simulink model "ROPOD_Control_SIM"  (R2017b)
settings: Solver=VariableStepAuto  StartTime=0.0  StopTime=inf  RelTol=1e-3
values from neighbouring files (symbols this model uses):
  AgentNumber = 1    [init_model.m]
  FFtheta_intia = 0    [init_model.m]
  FFxy_mass = 0*80    (= 0)    [init_model.m]
  flock_FFtheta_friction = 50    [init_model.m]
  flock_FFxy_friction = 100    [init_model.m]
  I_fhz_ddelta_cntr = 0    [init_model.m]
  I_fhz_dtheta_cntr = 0.3    [init_model.m]
  I_fhz_dtheta_flock_cntr = 0.1    [init_model.m]
  I_fhz_dvarphi_cntr = 0    [init_model.m]
  I_fhz_dxdy_cntr = 0.25    [init_model.m]
  I_fhz_dxdy_flock_cntr = 0.1    [init_model.m]
  K_gain_ddelta_cntr = 0.1    [init_model.m]
  K_gain_dtheta_cntr = 150    [init_model.m]
  K_gain_dtheta_flock_cntr = 100    [init_model.m]
  K_gain_dvarphi_cntr = 0.05    [init_model.m]
  K_gain_dxdy_cntr = 200    [init_model.m]
  K_gain_dxdy_flock_cntr = 200    [init_model.m]
  LL_wp_fhz_ddelta_cntr = 2    [init_model.m]
  LL_wp_fhz_dtheta_cntr = 20    [init_model.m]
  LL_wp_fhz_dtheta_flock_cntr = 20    [init_model.m]
  LL_wp_fhz_dvarphi_cntr = 10    [init_model.m]
  LL_wp_fhz_dxdy_cntr = 20    [init_model.m]
  LL_wp_fhz_dxdy_flock_cntr = 20    [init_model.m]
  LL_wz_fhz_ddelta_cntr = 2    [init_model.m]
  LL_wz_fhz_dtheta_cntr = 20    [init_model.m]
  LL_wz_fhz_dtheta_flock_cntr = 20    [init_model.m]
  LL_wz_fhz_dvarphi_cntr = 2    [init_model.m]
  LL_wz_fhz_dxdy_cntr = 20    [init_model.m]
  LL_wz_fhz_dxdy_flock_cntr = 20    [init_model.m]
  LPF_fhz_ddelta_cntr = 50    [init_model.m]
  LPF_fhz_ddelta_meas = 50    [init_model.m]
  LPF_fhz_dtheta_cntr = 100    [init_model.m]
  LPF_fhz_dtheta_flock_cntr = 40    [init_model.m]
  LPF_fhz_dvarphi_cntr = 50    [init_model.m]
  LPF_fhz_dvarphi_meas = 50    [init_model.m]
  LPF_fhz_dxdy_cntr = 100    [init_model.m]
  LPF_fhz_dxdy_flock_cntr = 40    [init_model.m]
  max_flock_acc_theta = 0.5    [init_model.m]
  max_flock_acc_xy = 0.5    [init_model.m]
  max_flock_vel_theta = 1.0    (= 1)    [init_model.m]
  max_flock_vel_xy = 1.0    (= 1)    [init_model.m]
  max_hw_tau = 7.0    (= 7)    [init_model.m]
  max_ropod_acc_theta = 1.6    [init_model.m]
  max_ropod_acc_xy = 2.0    (= 2)    [init_model.m]
  max_ropod_sw_force = 500    [init_model.m]
  max_ropod_sw_tau = 250    [init_model.m]
  max_ropod_vel_theta = 1.6    [init_model.m]
  max_ropod_vel_xy = 2.0    (= 2)    [init_model.m]
  max_sw_current = 10    [init_model.m]
  Nagents = 2    [init_model.m]
  Nwheels = 4    [Jqwl_numeric_function.m]    (also in S_matrix.m; extract_kinmodel_parameters.m; init_model.m; tau_optimal_dist_vec_fun.m)
  pivot_offs_sws = [0.0243    0.4689    0.3384    5.9050]    [init_model.m]
  ropod_kinmodel_pv = struct2array(ropod_kinmodel_param)    [set_ropod_KinModparams.m]
  ropod_position_inflock = [-1 0 3.1416]    [init_model.m]
  SW_COM1_ENABLE1 = hex2dec('0001')    [init_model.m]
  SW_COM1_ENABLE2 = hex2dec('0002')    [init_model.m]
  SW_COM1_MODE_TORQUE = bitshift(hex2dec('0000'),2)    [init_model.m]
  SW_COM1_MODE_VELOCITY = bitshift(hex2dec('0002'),2)    [init_model.m]
  SW_COM1_USE_TS = hex2dec('8000')    [init_model.m]
  sw_tau_2_current = 1/motor_physical_parameters.torqueconstant.value    [init_model.m]
  Tinit = 2    [init_model.m]
  Ts = 0.001    [init_model.m]
  Ts_MPC = 0.01    [init_model.m]
  Tsflck = 0.01    [init_model.m]
undefined symbols (not defined in the file or in its folder): acc_limit, accmax, b_cx, b_cy, b_rx, bus_size, comp_enable, Desired, DiscIntNeverNeededParam, Fcgain, gdis, k_cx, k_cy, live_tuning, m_robot, Nominal, Nominal_x, Nominal_y, offsets, portwidth, sizes, types, vel_limit, vmax1, vmax2
libraries: simulink x90, cstblocks x66, dspsigops x12, dspnetwork x4
(part 4 of 8)

== system ROPOD_Control_SIM/RopodTorqueDistribution/wheel vel cntr/Wheels Velocity controller ==
  dvarphi_error : Inport
  ena_w : Inport  Port=2
  platform_dvarphi_cntr_param : Inport  Port=3
  reset_int : Inport  Port=4
  Demux : Demux  Outputs=8
  Demux1 : Demux
  G_I_LL_LPF Controller1 : Subsystem
  G_I_LL_LPF Controller2 : Subsystem
  G_I_LL_LPF Controller3 : Subsystem
  G_I_LL_LPF Controller4 : Subsystem
  G_I_LL_LPF Controller5 : Subsystem
  G_I_LL_LPF Controller6 : Subsystem
  G_I_LL_LPF Controller7 : Subsystem
  G_I_LL_LPF Controller8 : Subsystem
  Mux : Mux  Inputs=8
  Mux1 : Mux  Inputs=8
  Product9 : Product
  varphi_tau_setp : Outport
  wires:
  Product9/1 -> Demux/1
  dvarphi_error/1 -> Product9/1
  [reset_int_cntr] -> G_I_LL_LPF Controller1/3(reset_integrator)
  Demux/1 -> G_I_LL_LPF Controller1/2(In)
  [param_dvarphi_cntr] -> G_I_LL_LPF Controller1/1(param)
  platform_dvarphi_cntr_param/1 -> [param_dvarphi_cntr]
  reset_int/1 -> [reset_int_cntr]
  [param_dvarphi_cntr] -> G_I_LL_LPF Controller2/1(param)
  [reset_int_cntr] -> G_I_LL_LPF Controller2/3(reset_integrator)
  Demux/2 -> G_I_LL_LPF Controller2/2(In)
  [reset_int_cntr] -> G_I_LL_LPF Controller4/3(reset_integrator)
  Demux/3 -> G_I_LL_LPF Controller3/2(In)
  Demux/4 -> G_I_LL_LPF Controller4/2(In)
  [param_dvarphi_cntr] -> G_I_LL_LPF Controller4/1(param)
  [param_dvarphi_cntr] -> G_I_LL_LPF Controller3/1(param)
  [reset_int_cntr] -> G_I_LL_LPF Controller3/3(reset_integrator)
  [param_dvarphi_cntr] -> G_I_LL_LPF Controller5/1(param)
  Demux/8 -> G_I_LL_LPF Controller8/2(In)
  [param_dvarphi_cntr] -> G_I_LL_LPF Controller7/1(param)
  [param_dvarphi_cntr] -> G_I_LL_LPF Controller8/1(param)
  [reset_int_cntr] -> G_I_LL_LPF Controller8/3(reset_integrator)
  [param_dvarphi_cntr] -> G_I_LL_LPF Controller6/1(param)
  [reset_int_cntr] -> G_I_LL_LPF Controller7/3(reset_integrator)
  Demux/6 -> G_I_LL_LPF Controller6/2(In)
  Demux/7 -> G_I_LL_LPF Controller7/2(In)
  [reset_int_cntr] -> G_I_LL_LPF Controller6/3(reset_integrator)
  [reset_int_cntr] -> G_I_LL_LPF Controller5/3(reset_integrator)
  Demux/5 -> G_I_LL_LPF Controller5/2(In)
  G_I_LL_LPF Controller1/1(Out) -> Mux/1
  G_I_LL_LPF Controller2/1(Out) -> Mux/2
  G_I_LL_LPF Controller4/1(Out) -> Mux/4
  G_I_LL_LPF Controller3/1(Out) -> Mux/3
  G_I_LL_LPF Controller5/1(Out) -> Mux/5
  G_I_LL_LPF Controller6/1(Out) -> Mux/6
  G_I_LL_LPF Controller7/1(Out) -> Mux/7
  G_I_LL_LPF Controller8/1(Out) -> Mux/8
  Mux/1 -> varphi_tau_setp/1
  ena_w/1 -> Demux1/1
  Demux1/1 -> Mux1/2, Mux1/1
  Demux1/2 -> Mux1/4, Mux1/3
  Demux1/3 -> Mux1/6, Mux1/5
  Demux1/4 -> Mux1/8, Mux1/7
  Mux1/1 -> Product9/2

== system ROPOD_Control_SIM/RopodVelocityController/Platorm Velocity controller/G_I_LL_LPF Controller_X ==
  param : Inport
  In : Inport  Port=2
  reset_integrator : Inport  Port=3
  Bus Selector : BusSelector  OutputSignals=P_gain,I_freq_hz,LL_zero_fhz,LL_pole_fhz,LPF_fhz
  Discrete Varying Lowpass3 : cstblocks/Linear Parameter Varying/Discrete Varying Lowpass  N=1  w0=0  Ts=Ts
      settings: SourceProductName=Control System Toolbox  SourceProductBaseCode=CT
  Gain2 : Gain  Gain=2*pi
  Product5 : Product
  Shapeit Integrator (Tustin) : Subsystem
  Shapeit Lead-Lag (Tustin) : Subsystem
  Out : Outport
  wires:
  Gain2/1 -> Discrete Varying Lowpass3/2
  Product5/1 -> Shapeit Integrator (Tustin)/1(In)
  Discrete Varying Lowpass3/1 -> Out/1
  Shapeit Integrator (Tustin)/1(Out) -> Shapeit Lead-Lag (Tustin)/1(In)
  Bus Selector/1 -> Product5/2  "<P_gain>"
  Bus Selector/2 -> Shapeit Integrator (Tustin)/2(I_fhz)  "<I_freq_hz>"
  param/1 -> Bus Selector/1
  Bus Selector/5 -> Gain2/1  "<LPF_fhz>"
  Bus Selector/4 -> Shapeit Lead-Lag (Tustin)/3(fp)  "<LL_pole_fhz>"
  reset_integrator/1 -> Shapeit Integrator (Tustin)/3(reset)
  Bus Selector/3 -> Shapeit Lead-Lag (Tustin)/2(fz)  "<LL_zero_fhz>"
  Shapeit Lead-Lag (Tustin)/1(Out) -> Discrete Varying Lowpass3/1
  In/1 -> Product5/1

== system ROPOD_Control_SIM/RopodVelocityController/Platorm Velocity controller/G_I_LL_LPF Controller_Y ==
  param : Inport
  In : Inport  Port=2
  reset_integrator : Inport  Port=3
  Bus Selector : BusSelector  OutputSignals=P_gain,I_freq_hz,LL_zero_fhz,LL_pole_fhz,LPF_fhz
  Discrete Varying Lowpass3 : cstblocks/Linear Parameter Varying/Discrete Varying Lowpass  N=1  w0=0  Ts=Ts
      settings: SourceProductName=Control System Toolbox  SourceProductBaseCode=CT
  Gain2 : Gain  Gain=2*pi
  Product5 : Product
  Shapeit Integrator (Tustin) : Subsystem
  Shapeit Lead-Lag (Tustin) : Subsystem
  Out : Outport
  wires:
  Gain2/1 -> Discrete Varying Lowpass3/2
  Product5/1 -> Shapeit Integrator (Tustin)/1(In)
  Discrete Varying Lowpass3/1 -> Out/1
  Shapeit Integrator (Tustin)/1(Out) -> Shapeit Lead-Lag (Tustin)/1(In)
  Bus Selector/1 -> Product5/2  "<P_gain>"
  Bus Selector/2 -> Shapeit Integrator (Tustin)/2(I_fhz)  "<I_freq_hz>"
  param/1 -> Bus Selector/1
  Bus Selector/5 -> Gain2/1  "<LPF_fhz>"
  Bus Selector/4 -> Shapeit Lead-Lag (Tustin)/3(fp)  "<LL_pole_fhz>"
  reset_integrator/1 -> Shapeit Integrator (Tustin)/3(reset)
  Bus Selector/3 -> Shapeit Lead-Lag (Tustin)/2(fz)  "<LL_zero_fhz>"
  Shapeit Lead-Lag (Tustin)/1(Out) -> Discrete Varying Lowpass3/1
  In/1 -> Product5/1

== system ROPOD_Control_SIM/RopodVelocityController/Platorm Velocity controller/G_I_LL_LPF Controller_theta ==
  param : Inport
  In : Inport  Port=2
  reset_integrator : Inport  Port=3
  Bus Selector : BusSelector  OutputSignals=P_gain,I_freq_hz,LL_zero_fhz,LL_pole_fhz,LPF_fhz
  Discrete Varying Lowpass3 : cstblocks/Linear Parameter Varying/Discrete Varying Lowpass  N=1  w0=0  Ts=Ts
      settings: SourceProductName=Control System Toolbox  SourceProductBaseCode=CT
  Gain2 : Gain  Gain=2*pi
  Product5 : Product
  Shapeit Integrator (Tustin) : Subsystem
  Shapeit Lead-Lag (Tustin) : Subsystem
  Out : Outport
  wires:
  Gain2/1 -> Discrete Varying Lowpass3/2
  Product5/1 -> Shapeit Integrator (Tustin)/1(In)
  Discrete Varying Lowpass3/1 -> Out/1
  Shapeit Integrator (Tustin)/1(Out) -> Shapeit Lead-Lag (Tustin)/1(In)
  Bus Selector/1 -> Product5/2  "<P_gain>"
  Bus Selector/2 -> Shapeit Integrator (Tustin)/2(I_fhz)  "<I_freq_hz>"
  param/1 -> Bus Selector/1
  Bus Selector/5 -> Gain2/1  "<LPF_fhz>"
  Bus Selector/4 -> Shapeit Lead-Lag (Tustin)/3(fp)  "<LL_pole_fhz>"
  reset_integrator/1 -> Shapeit Integrator (Tustin)/3(reset)
  Bus Selector/3 -> Shapeit Lead-Lag (Tustin)/2(fz)  "<LL_zero_fhz>"
  Shapeit Lead-Lag (Tustin)/1(Out) -> Discrete Varying Lowpass3/1
  In/1 -> Product5/1

== system ROPOD_Control_SIM/Subsystem1/Compliant control/Ground [3,1] ==
  Ground : Ground
  Ground1 : Ground
  Ground2 : Ground
  Mux : Mux  Inputs=3
  Out1 : Outport
  wires:
  Ground1/1 -> Mux/2
  Mux/1 -> Out1/1
  Ground2/1 -> Mux/3
  Ground/1 -> Mux/1

== system ROPOD_Control_SIM/Subsystem1/Compliant control/Ground [3,1]1 ==
  Ground : Ground
  Ground1 : Ground
  Ground2 : Ground
  Mux : Mux  Inputs=3
  Out1 : Outport
  wires:
  Ground1/1 -> Mux/2
  Mux/1 -> Out1/1
  Ground2/1 -> Mux/3
  Ground/1 -> Mux/1

== system ROPOD_Control_SIM/Subsystem1/Compliant control/Ground [3,1]2 ==
  Ground : Ground
  Ground1 : Ground
  Ground2 : Ground
  Mux : Mux  Inputs=3
  Out1 : Outport
  wires:
  Ground1/1 -> Mux/2
  Mux/1 -> Out1/1
  Ground2/1 -> Mux/3
  Ground/1 -> Mux/1

== system ROPOD_Control_SIM/Subsystem1/Compliant control/Impedance ==
  X0 : Inport
  Y0 : Inport  Port=2
  theta0i : Inport  Port=3
  x : Inport  Port=4
  y : Inport  Port=5
  theta : Inport  Port=6
  Fext : Inport  Port=7
  motion tuning bus : Inport  Port=8
  Bus decoder : S-Function  FunctionName=sf_bus_decode  Parameters=sizes,offsets,portwidth,types,bus_size  SFunctionDeploymentMode=off  EnableBusSupport=off  mask(Decode bus variables.){bus_name=tunable_pardata_motion_bus, var_name01=off, var_name02=off, var_name03=off, var_name04=off, var_name05=off, var_name06=off, var_name07=off, var_name08=off, var_name09=off, var_name10=off, var_name11=off, var_name12=off, var_name13=off, var_name14=off, var_name15=off, var_name16=off, var_name17=off, var_name18=off, var_name19=off, var_name20=off, var_name21=off, var_name22=off, var_name23=off, var_name24=off, var_name25=off, var_name26=off, var_name27=off, var_name28=off, var_name29=off, var_name30=off, var_name31=off, var_name32=off, var_name33=off, var_name34=off, var_name35=off, var_name36=off, var_name37=off, var_name38=off, var_name39=off, var_name40=off, var_name41=off, var_name42=off, var_name43=off, var_name44=off, var_name45=off, var_name46=off, var_name47=off, var_name48=off, var_name49=off, var_name50=off, var_name51=off, var_name52=off, var_name53=off, var_name54=off, var_name55=off, var_name56=off, var_name57=off, var_name58=off, var_name59=off, var_name60=off, var_name61=off, var_name62=off, var_name63=off, var_name64=off, var_name65=off, var_name66=off, var_name67=off, var_name68=off, var_name69=off, var_name70=off, var_name71=off, var_name72=off, var_name73=off, var_name74=off, var_name75=off, var_name76=off, var_name77=off, var_name78=off, var_name79=off, var_name80=off, var_name81=off, var_name82=off, var_name83=off, var_name84=off, var_name85=on, var_name86=on, var_name87=on, var_name88=on, var_name89=off, var_name90=off, var_name91=off, var_name92=off, var_name93=off, var_name94=off, var_name95=off, var_name96=off, var_name97=off, var_name98=off, var_name99=off, var_name100=off, selected_bus=tunable_pardata_motion_bus, var_ids=113,128,5,6,8,9,92,93,11,12,56,14,15,57,40,41,42,43,44,45,58,74,75,76,77,78,73,20,52,125,129,23,95,91,100,101,89,90,60,24,69,70,81,82,88,98,126,131,134,26,120,27,28,29,30,130,135,103,31,32,33,34,35,136,36,37,38,39,83,99,111,105,106,110,109,107,108,112,114,115,116,117,118,132,137,138,139,140,, checked_var_ids=139,138,137,140,}
      mask prompts: bus_name "Name of bus"; var_name01 "deceleration_gain"; var_name02 "deceleration_gain_hb"; var_name03 "SF_v_max_move"; var_name04 "SF_v_max_dribble"; var_name05 "SF_a_max_move"; var_name06 "SF_a_max_dribble"; var_name07 "SF_a_max_passes"; var_name08 "SF_a_max_push"; var_name09 "SF_v_max_rotate_move"; var_name10 "SF_v_max_rotate_dribble"; var_name11 "SF_v_max_rotate_aim_refbox"; var_name12 "SF_a_max_rotate_move"; var_name13 "SF_a_max_rotate_dribble"; var_name14 "SF_a_max_rotate_aim_refbox"; var_name15 "SF_v_max_x_keeper"; var_name16 "SF_v_max_y_keeper"; var_name17 "SF_a_max_x_keeper"; var_name18 "SF_a_max_y_keeper"; var_name19 "SF_v_max_rotate_keeper"; var_name20 "SF_a_max_rotate_keeper"; var_name21 "SF_perc_torque_front_wheels"; var_name22 "TPPP_val0v"; var_name23 "TPPP_val0a"; var_name24 "TPPP_err0"; var_name25 "TPPP_val1"; var_name26 "TPPP_err1"; var_name27 "SF_shock_bound"; var_name28 "BH_AngleReference"; var_name29 "BH_AngleReferenceKick"; var_name30 "BH_AngleReferenceScrum"; var_name31 "BH_AngleReferenceShock"; var_name32 "BH_VelocityReferenceNoBall"; var_name33 "BH_VelReferenceNoBallLow"; var_name34 "BH_VelReferenceNoBallHigh"; var_name35 "BH_VelRefStupidHumanDribble"; var_name36 "BH_StupidHumanDribbleOnOff"; var_name37 "BH_CatchingTime"; var_name38 "BH_FF_base_factor"; var_name39 "BH_AddRetractForwardDribble"; var_name40 "BH_AddRetractBackwardDribble"; var_name41 "BH_AddRetractSidewaysBackArm"; var_name42 "BH_AddRetractSidewaysFrontArm"; var_name43 "BH_PGain_CAngle"; var_name44 "BH_PGain_CVel"; var_name45 "BH_PGain_CVel_catching"; var_name46 "BH_use_scrumhandler"; var_name47 "BH_Enable_Logging"; var_name48 "BH_CRK_Cnt_Thresh"; var_name49 "BH_AimAngleErr_BeforeRetract"; var_name50 "K_retract_ball_timeout_ms"; var_name51 "K_retract_ball_time_penalty_ms"; var_name52 "K_basis_value_lob"; var_name53 "K_rate_value_lob"; var_name54 "K_basis_value_pass"; var_name55 "K_rate_value_pass"; var_name56 "K_game2velmap"; var_name57 "K_KinectLob_angle_subtract"; var_name58 "K_PassTimeGain_dyn_Pass"; var_name59 "K_maximum_value_flat"; var_name60 "K_angle_flat_shot"; var_name61 "K_velocity_gain_lob"; var_name62 "K_wait_time_during_aim_in_s"; var_name63 "K_use_demo_goal"; var_name64 "K_do_large_goal_holes_demo"; var_name65 "K_width_holes"; var_name66 "K_height_hole2"; var_name67 "K_height_hole3"; var_name68 "K_FFBallSpeedOnAimTarget"; var_name69 "K_FFBallSpeedOnAimTargetPass"; var_name70 "K_FFBallSpeedOnAimTargetLob"; var_name71 "K_shoot_when_retracted"; var_name72 "SF_brake_gain_target_turtle"; var_name73 "SF_brake_gain_reverse_turtle"; var_name74 "SF_brake_gain_target_pass"; var_name75 "SF_brake_gain_reverse_pass"; var_name76 "SF_brake_gain_target_keeper"; var_name77 "SF_brake_gain_reverse_keeper"; var_name78 "SF_ball2robotdist_for_rotate"; var_name79 "lobExtraDistanceComp_Turtle2"; var_name80 "lobExtraDistanceComp_Turtle3"; var_name81 "lobExtraDistanceComp_Turtle4"; var_name82 "lobExtraDistanceComp_Turtle5"; var_name83 "lobExtraDistanceComp_Turtle6"; var_name84 "LED_mainswitch"; var_name85 "Desired_Mass"; var_name86 "Desired_Damping"; var_name87 "Desired_Friction"; var_name88 "Vel_limit"; var_name89 "0"; var_name90 "0"; var_name91 "0"; var_name92 "0"; var_name93 "0"; var_name94 "0"; var_name95 "0"; var_name96 "0"; var_name97 "0"; var_name98 "0"; var_name99 "0"; var_name100 "0"; selected_bus "memory variable"; var_ids "memory variable"; checked_var_ids "memory variable"
      mask help:
      | Bus decoder to obtain values of bus variables.
      | Busses can be editted and created using the busmanager. Note that deleting input variables of this bus assigner will mix the inputs.
      mask init:
      | [bus_size, types, portwidth, sizes, offsets] = mask_sf_bus_decode('init');
      mask TypeOptions bus_name: <Select bus> | TRCbus | motionbus | teambus | visionbus | tunable_pardata_motion_bus | tunable_pardata_vision_bus | tunable_pardata_strategy_bus | actionsbus | controlbus | strategybus | sensorfusionbus | refboxparamsbus | tunable_pardata_worldmodel_bus
      mask Callback bus_name: mask_sf_bus_decode('init');
      mask Display:
      | port_label('output',1,'Desired_Friction');
      | port_label('output',2,'Desired_Damping');
      | port_label('output',3,'Desired_Mass');
      | port_label('output',4,'Vel_limit');
      | port_label('input',1,'tunable_pardata_motion_bus')
  Demux : Demux  Outputs=3
  Demux1 : Demux  Outputs=3
  Demux3 : Demux  Outputs=3
  Impedance control : MATLAB Function  TreatAsAtomicUnit=on
  Mux : Mux
  Mux1 : Mux  Inputs=2
  Mux3 : Mux  Inputs=2
  Mux5 : Mux  Inputs=2
  Selector : Selector  InputPortWidth=4  IndexOptions=Index vector (dialog)  Indices=[3 2 1 4]  OutputSizes=1
  Terminator1 : Terminator
  Terminator2 : Terminator
  Terminator5 : Terminator
  To Workspace2 : ToWorkspace  VariableName=live_param  SampleTime=-1
  Transfer Fcn1 : TransferFcn  Numerator=[gdis]  Denominator=[1 gdis]
  Transfer Fcn2 : TransferFcn  Numerator=[gdis]  Denominator=[1 gdis]
  Transfer Fcn4 : TransferFcn  Numerator=[gdis]  Denominator=[1 gdis]
  Imp_force : Outport
  wires:
  y/1 -> Demux/1
  Fext/1 -> Impedance control/7(Fext)
  Impedance control/1(F) -> Imp_force/1
  Demux/2 -> Transfer Fcn4/1
  Demux/1 -> Mux3/1
  Demux/3 -> Terminator2/1
  Transfer Fcn4/1 -> Mux3/2
  Mux3/1 -> Impedance control/5(q2)
  X0/1 -> Impedance control/1(x0i)
  x/1 -> Demux1/1
  Demux1/2 -> Transfer Fcn1/1
  Demux1/1 -> Mux1/1
  Demux1/3 -> Terminator1/1
  Transfer Fcn1/1 -> Mux1/2
  Mux1/1 -> Impedance control/4(q1)
  Y0/1 -> Impedance control/2(y0i)
  theta/1 -> Demux3/1
  Demux3/2 -> Transfer Fcn2/1
  Demux3/1 -> Mux5/1
  Demux3/3 -> Terminator5/1
  Transfer Fcn2/1 -> Mux5/2
  Mux5/1 -> Impedance control/6(q3)
  Bus decoder/1 -> Mux/1
  Bus decoder/2 -> Mux/2
  Bus decoder/3 -> Mux/3
  motion tuning bus/1 -> Bus decoder/1
  Selector/1 -> Impedance control/8(params_xy), To Workspace2/1
  Mux/1 -> Selector/1
  theta0i/1 -> Impedance control/3(theta0i)
  Bus decoder/4 -> Mux/4

== system ROPOD_Control_SIM/Subsystem1/Observer/DOB3 ==
  Control input : Inport
  x : Inport  Port=2
  y : Inport  Port=3
  theta : Inport  Port=4
  Abs : Abs
  Acc_limit : Subsystem
  Constant : Constant
  Dead Zone : DeadZone  LowerValue=-0.01  UpperValue=0.01  SaturateOnIntegerOverflow=on
  Divide : Product  Inputs=/*  SaturateOnIntegerOverflow=on  RndMeth=Zero
  Gain : Gain  Gain=Nominal.mass
  Gain1 : Gain  Gain=Nominal.damping
  Gain2 : Gain  Gain=Nominal.Fd
  Gain3 : Gain  Gain=[1;1;0.2]
  Gain4 : Gain  Gain=40
  Low-Pass1 : Subsystem
  Low-Pass2 : Subsystem
  Low-Pass3 : Subsystem
  Math Function1 : Math  Operator=square  SaturateOnIntegerOverflow=on
  Mux2 : Mux  Inputs=3
  Mux3 : Mux  Inputs=3
  Product : Product
  Selector1 : Selector  InputPortWidth=3  IndexOptions=Index vector (dialog)  Indices=[3]  OutputSizes=1
  Selector2 : Selector  InputPortWidth=3  IndexOptions=Index vector (dialog)  Indices=[3]  OutputSizes=1
  Selector3 : Selector  InputPortWidth=3  IndexOptions=Index vector (dialog)  Indices=[2]  OutputSizes=1
  Selector4 : Selector  InputPortWidth=3  IndexOptions=Index vector (dialog)  Indices=[2]  OutputSizes=1
  Selector6 : Selector  InputPortWidth=3  IndexOptions=Index vector (dialog)  Indices=[3]  OutputSizes=1
  Selector7 : Selector  InputPortWidth=3  IndexOptions=Index vector (dialog)  Indices=[2]  OutputSizes=1
  Sin : Trigonometry  Operator=tanh
  Sqrt1 : Sqrt  SaturateOnIntegerOverflow=on
  Sum : Sum  Inputs=+++
  Sum of Elements1 : Sum  Inputs=+
  Sum3 : Sum  Inputs=-+|
  Switch : Switch  Criteria=u2 ~= 0
  To Workspace2 : ToWorkspace  VariableName=acc  SampleTime=-1
  Estimated disturbance : Outport
  wires:
  Gain/1 -> Sum/1
  Mux2/1 -> Low-Pass1/1(In1)
  Mux3/1 -> Low-Pass2/1(In1)
  Sum/1 -> Sum3/2
  Gain1/1 -> Sum/2
  x/1 -> Selector3/1, Selector1/1
  Math Function1/1 -> Sum of Elements1/1
  Sum of Elements1/1 -> Sqrt1/1
  y/1 -> Selector2/1, Selector4/1
  Selector1/1 -> Mux2/1
  Selector2/1 -> Mux2/2
  Selector3/1 -> Mux3/1
  Selector4/1 -> Mux3/2
  Control input/1 -> Low-Pass3/1(In1)
  Sum3/1 -> Estimated disturbance/1
  Dead Zone/1 -> Gain1/1, Gain3/1
  Low-Pass3/1(Out1) -> Sum3/1
  Low-Pass2/1(Out1) -> Dead Zone/1
  theta/1 -> Selector7/1, Selector6/1
  Selector6/1 -> Mux2/3
  Selector7/1 -> Mux3/3
  Gain2/1 -> Sum/3
  Product/1 -> Gain2/1
  Divide/1 -> Abs/1
  Gain4/1 -> Sin/1
  Sin/1 -> Product/2
  Abs/1 -> Product/1
  Sqrt1/1 -> Switch/1, Switch/2
  Switch/1 -> Divide/1
  Constant/1 -> Switch/3
  Low-Pass1/1(Out1) -> Acc_limit/1(acc_in)
  Acc_limit/1(acc_out) -> To Workspace2/1, Gain/1
  Gain3/1 -> Gain4/1, Divide/2, Math Function1/1

== system ROPOD_Control_SIM/Subsystem1/Observer/DOB_x ==
  Control input : Inport
  System states : Inport  Port=2
  Demux : Demux  Outputs=3
  Gain : Gain  Gain=Nominal_x.mass
  Gain1 : Gain  Gain=Nominal_x.damping
  Gain2 : Gain  Gain=Nominal_x.Fd
  Gain4 : Gain  Gain=40
  Sin : Trigonometry  Operator=tanh
  Sum : Sum  Inputs=+++
  Sum3 : Sum  Inputs=-+|
  Terminator : Terminator
  Transfer Fcn3 : TransferFcn  Numerator=[gdis]  Denominator=[1 gdis]
  Transfer Fcn4 : TransferFcn  Numerator=[gdis]  Denominator=[1 gdis]
  Estimated disturbance : Outport
  wires:
  Sum/1 -> Sum3/2
  Gain1/1 -> Sum/2
  Control input/1 -> Sum3/1
  System states/1 -> Demux/1
  Sin/1 -> Gain2/1
  Gain4/1 -> Sin/1
  Gain2/1 -> Sum/1
  Sum3/1 -> Transfer Fcn4/1
  Transfer Fcn4/1 -> Transfer Fcn3/1
  Demux/3 -> Gain/1
  Demux/2 -> Gain4/1, Gain1/1
  Transfer Fcn3/1 -> Estimated disturbance/1
  Demux/1 -> Terminator/1
  Gain/1 -> Sum/3

== system ROPOD_Control_SIM/Subsystem1/Observer/DOB_y ==
  Control input : Inport
  System states : Inport  Port=2
  Demux : Demux  Outputs=3
  Gain : Gain  Gain=Nominal_y.mass
  Gain1 : Gain  Gain=Nominal_y.damping
  Gain2 : Gain  Gain=Nominal_y.Fd
  Gain4 : Gain  Gain=40
  Sin : Trigonometry  Operator=tanh
  Sum : Sum  Inputs=+++
  Sum3 : Sum  Inputs=-+|
  Terminator : Terminator
  Transfer Fcn3 : TransferFcn  Numerator=[gdis]  Denominator=[1 gdis]
  Transfer Fcn4 : TransferFcn  Numerator=[gdis]  Denominator=[1 gdis]
  Estimated disturbance : Outport
  wires:
  Sum/1 -> Sum3/2
  Gain1/1 -> Sum/2
  Control input/1 -> Sum3/1
  System states/1 -> Demux/1
  Sin/1 -> Gain2/1
  Gain4/1 -> Sin/1
  Gain2/1 -> Sum/1
  Sum3/1 -> Transfer Fcn4/1
  Transfer Fcn4/1 -> Transfer Fcn3/1
  Demux/3 -> Gain/1
  Demux/2 -> Gain4/1, Gain1/1
  Transfer Fcn3/1 -> Estimated disturbance/1
  Demux/1 -> Terminator/1
  Gain/1 -> Sum/3

== system ROPOD_Control_SIM/Subsystem2/Bumper_system/Lo-Pass filter1 ==
  s_data : Inport
  Constant : Constant  Value=2*pi*0.8
  Demux : Demux  Outputs=8
  Discrete Varying Lowpass{1..8} (8 alike) : cstblocks/Linear Parameter Varying/Discrete Varying Lowpass  N=1  w0=0  Ts=Ts_MPC
      settings: SourceProductName=Control System Toolbox  SourceProductBaseCode=CT
  Mux : Mux  Inputs=8
  Rate Transition{,1..7} (8 alike) : RateTransition  OutPortSampleTime=Ts_MPC
  Transfer Fcn1 : TransferFcn  Commented=on  Denominator=[(1/(2*pi*0.8)) 1]
  Filterd_s_data : Outport
  wires:
  Mux/1 -> Filterd_s_data/1
  Demux/6 -> Discrete Varying Lowpass5/1
  Demux/5 -> Discrete Varying Lowpass6/1
  Demux/3 -> Discrete Varying Lowpass3/1
  Demux/2 -> Discrete Varying Lowpass1/1
  Demux/1 -> Discrete Varying Lowpass2/1
  s_data/1 -> Demux/1
  Demux/7 -> Discrete Varying Lowpass7/1
  Demux/8 -> Discrete Varying Lowpass8/1
  Demux/4 -> Discrete Varying Lowpass4/1
  Discrete Varying Lowpass2/1 -> Rate Transition/1
  Discrete Varying Lowpass1/1 -> Rate Transition1/1
  Discrete Varying Lowpass3/1 -> Rate Transition2/1
  Discrete Varying Lowpass4/1 -> Rate Transition3/1
  Discrete Varying Lowpass6/1 -> Rate Transition4/1
  Discrete Varying Lowpass5/1 -> Rate Transition5/1
  Discrete Varying Lowpass7/1 -> Rate Transition6/1
  Discrete Varying Lowpass8/1 -> Rate Transition7/1
  Constant/1 -> Discrete Varying Lowpass1/2, Discrete Varying Lowpass3/2, Discrete Varying Lowpass4/2, Discrete Varying Lowpass6/2, Discrete Varying Lowpass5/2, Discrete Varying Lowpass8/2, Discrete Varying Lowpass7/2, Discrete Varying Lowpass2/2
  Rate Transition/1 -> Mux/1
  Rate Transition1/1 -> Mux/2
  Rate Transition3/1 -> Mux/4
  Rate Transition2/1 -> Mux/3
  Rate Transition7/1 -> Mux/8
  Rate Transition4/1 -> Mux/5
  Rate Transition5/1 -> Mux/6
  Rate Transition6/1 -> Mux/7

== system ROPOD_Control_SIM/Subsystem2/Bumper_system/Lo-Pass filter2 ==
  s_data : Inport
  Constant : Constant  Value=2*pi*0.8
  Demux : Demux  Outputs=8
  Discrete Varying Lowpass{1..8} (8 alike) : cstblocks/Linear Parameter Varying/Discrete Varying Lowpass  N=1  w0=0  Ts=Ts_MPC
      settings: SourceProductName=Control System Toolbox  SourceProductBaseCode=CT
  Mux : Mux  Inputs=8
  Rate Transition{,1..7} (8 alike) : RateTransition  OutPortSampleTime=Ts_MPC
  Transfer Fcn1 : TransferFcn  Commented=on  Denominator=[(1/(2*pi*0.8)) 1]
  Filterd_s_data : Outport
  wires:
  Mux/1 -> Filterd_s_data/1
  Demux/6 -> Discrete Varying Lowpass5/1
  Demux/5 -> Discrete Varying Lowpass6/1
  Demux/3 -> Discrete Varying Lowpass3/1
  Demux/2 -> Discrete Varying Lowpass1/1
  Demux/1 -> Discrete Varying Lowpass2/1
  s_data/1 -> Demux/1
  Demux/7 -> Discrete Varying Lowpass7/1
  Demux/8 -> Discrete Varying Lowpass8/1
  Demux/4 -> Discrete Varying Lowpass4/1
  Discrete Varying Lowpass2/1 -> Rate Transition/1
  Discrete Varying Lowpass1/1 -> Rate Transition1/1
  Discrete Varying Lowpass3/1 -> Rate Transition2/1
  Discrete Varying Lowpass4/1 -> Rate Transition3/1
  Discrete Varying Lowpass6/1 -> Rate Transition4/1
  Discrete Varying Lowpass5/1 -> Rate Transition5/1
  Discrete Varying Lowpass7/1 -> Rate Transition6/1
  Discrete Varying Lowpass8/1 -> Rate Transition7/1
  Constant/1 -> Discrete Varying Lowpass1/2, Discrete Varying Lowpass3/2, Discrete Varying Lowpass4/2, Discrete Varying Lowpass6/2, Discrete Varying Lowpass5/2, Discrete Varying Lowpass8/2, Discrete Varying Lowpass7/2, Discrete Varying Lowpass2/2
  Rate Transition/1 -> Mux/1
  Rate Transition1/1 -> Mux/2
  Rate Transition3/1 -> Mux/4
  Rate Transition2/1 -> Mux/3
  Rate Transition7/1 -> Mux/8
  Rate Transition4/1 -> Mux/5
  Rate Transition5/1 -> Mux/6
  Rate Transition6/1 -> Mux/7

== system ROPOD_Control_SIM/Subsystem2/Bumper_system/Lo-Pass filter3 ==
  s_data : Inport
  Constant : Constant  Value=2*pi*0.8
  Demux : Demux  Outputs=8
  Discrete Varying Lowpass{1..8} (8 alike) : cstblocks/Linear Parameter Varying/Discrete Varying Lowpass  N=1  w0=0  Ts=Ts_MPC
      settings: SourceProductName=Control System Toolbox  SourceProductBaseCode=CT
  Mux : Mux  Inputs=8
  Rate Transition{,1..7} (8 alike) : RateTransition  OutPortSampleTime=Ts_MPC
  Transfer Fcn1 : TransferFcn  Commented=on  Denominator=[(1/(2*pi*0.8)) 1]
  Filterd_s_data : Outport
  wires:
  Mux/1 -> Filterd_s_data/1
  Demux/6 -> Discrete Varying Lowpass5/1
  Demux/5 -> Discrete Varying Lowpass6/1
  Demux/3 -> Discrete Varying Lowpass3/1
  Demux/2 -> Discrete Varying Lowpass1/1
  Demux/1 -> Discrete Varying Lowpass2/1
  s_data/1 -> Demux/1
  Demux/7 -> Discrete Varying Lowpass7/1
  Demux/8 -> Discrete Varying Lowpass8/1
  Demux/4 -> Discrete Varying Lowpass4/1
  Discrete Varying Lowpass2/1 -> Rate Transition/1
  Discrete Varying Lowpass1/1 -> Rate Transition1/1
  Discrete Varying Lowpass3/1 -> Rate Transition2/1
  Discrete Varying Lowpass4/1 -> Rate Transition3/1
  Discrete Varying Lowpass6/1 -> Rate Transition4/1
  Discrete Varying Lowpass5/1 -> Rate Transition5/1
  Discrete Varying Lowpass7/1 -> Rate Transition6/1
  Discrete Varying Lowpass8/1 -> Rate Transition7/1
  Constant/1 -> Discrete Varying Lowpass1/2, Discrete Varying Lowpass3/2, Discrete Varying Lowpass4/2, Discrete Varying Lowpass6/2, Discrete Varying Lowpass5/2, Discrete Varying Lowpass8/2, Discrete Varying Lowpass7/2, Discrete Varying Lowpass2/2
  Rate Transition/1 -> Mux/1
  Rate Transition1/1 -> Mux/2
  Rate Transition3/1 -> Mux/4
  Rate Transition2/1 -> Mux/3
  Rate Transition7/1 -> Mux/8
  Rate Transition4/1 -> Mux/5
  Rate Transition5/1 -> Mux/6
  Rate Transition6/1 -> Mux/7

== system ROPOD_Control_SIM/Subsystem2/Bumper_system/Lo-Pass filter4 ==
  s_data : Inport
  Constant : Constant  Value=2*pi*0.8
  Demux : Demux  Outputs=8
  Discrete Varying Lowpass{1..8} (8 alike) : cstblocks/Linear Parameter Varying/Discrete Varying Lowpass  N=1  w0=0  Ts=Ts_MPC
      settings: SourceProductName=Control System Toolbox  SourceProductBaseCode=CT
  Mux : Mux  Inputs=8
  Rate Transition{,1..7} (8 alike) : RateTransition  OutPortSampleTime=Ts_MPC
  Transfer Fcn1 : TransferFcn  Commented=on  Denominator=[(1/(2*pi*0.8)) 1]
  Filterd_s_data : Outport
  wires:
  Mux/1 -> Filterd_s_data/1
  Demux/6 -> Discrete Varying Lowpass5/1
  Demux/5 -> Discrete Varying Lowpass6/1
  Demux/3 -> Discrete Varying Lowpass3/1
  Demux/2 -> Discrete Varying Lowpass1/1
  Demux/1 -> Discrete Varying Lowpass2/1
  s_data/1 -> Demux/1
  Demux/7 -> Discrete Varying Lowpass7/1
  Demux/8 -> Discrete Varying Lowpass8/1
  Demux/4 -> Discrete Varying Lowpass4/1
  Discrete Varying Lowpass2/1 -> Rate Transition/1
  Discrete Varying Lowpass1/1 -> Rate Transition1/1
  Discrete Varying Lowpass3/1 -> Rate Transition2/1
  Discrete Varying Lowpass4/1 -> Rate Transition3/1
  Discrete Varying Lowpass6/1 -> Rate Transition4/1
  Discrete Varying Lowpass5/1 -> Rate Transition5/1
  Discrete Varying Lowpass7/1 -> Rate Transition6/1
  Discrete Varying Lowpass8/1 -> Rate Transition7/1
  Constant/1 -> Discrete Varying Lowpass1/2, Discrete Varying Lowpass3/2, Discrete Varying Lowpass4/2, Discrete Varying Lowpass6/2, Discrete Varying Lowpass5/2, Discrete Varying Lowpass8/2, Discrete Varying Lowpass7/2, Discrete Varying Lowpass2/2
  Rate Transition/1 -> Mux/1
  Rate Transition1/1 -> Mux/2
  Rate Transition3/1 -> Mux/4
  Rate Transition2/1 -> Mux/3
  Rate Transition7/1 -> Mux/8
  Rate Transition4/1 -> Mux/5
  Rate Transition5/1 -> Mux/6
  Rate Transition6/1 -> Mux/7

== system ROPOD_Control_SIM/Subsystem2/Bumper_system/cal ==
  In1 : Inport
  Calibration1 : MATLAB Function  TreatAsAtomicUnit=on  SystemSampleTime=Ts_MPC
  Memory2 : Memory  InitialCondition=1  InheritSampleTime=on
  Memory3 : Memory  InheritSampleTime=on
  Out1 : Outport
  wires:
  Calibration1/2(i) -> Memory2/1
  Memory2/1 -> Calibration1/2(sample)
  Memory3/1 -> Calibration1/3(data)
  In1/1 -> Calibration1/1(angle)
  Calibration1/1(cal_angle) -> Out1/1
  Calibration1/3(data_out) -> Memory3/1

== system ROPOD_Control_SIM/Subsystem2/Bumper_system/cal1 ==
  In1 : Inport
  Calibration1 : MATLAB Function  TreatAsAtomicUnit=on
  Memory2 : Memory  InitialCondition=1  InheritSampleTime=on
  Memory3 : Memory  InheritSampleTime=on
  Out2 : Outport
  Out1 : Outport  Port=2
  wires:
  Calibration1/4(data_out) -> Memory3/1
  Calibration1/2(cal_angle) -> Out1/1
  In1/1 -> Calibration1/1(angle)
  Memory3/1 -> Calibration1/3(data)
  Memory2/1 -> Calibration1/2(sample)
  Calibration1/3(i) -> Memory2/1
  Calibration1/1(cal_done) -> Out2/1

== system ROPOD_Control_SIM/Subsystem2/Bumper_system/cal2 ==
  In1 : Inport
  Calibration1 : MATLAB Function  TreatAsAtomicUnit=on  SystemSampleTime=Ts_MPC
  Memory2 : Memory  InitialCondition=1  InheritSampleTime=on
  Memory3 : Memory  InheritSampleTime=on
  Out1 : Outport
  wires:
  Calibration1/2(i) -> Memory2/1
  Memory2/1 -> Calibration1/2(sample)
  Memory3/1 -> Calibration1/3(data)
  In1/1 -> Calibration1/1(angle)
  Calibration1/1(cal_angle) -> Out1/1
  Calibration1/3(data_out) -> Memory3/1

== system ROPOD_Control_SIM/Subsystem2/Bumper_system/cal3 ==
  In1 : Inport
  Calibration1 : MATLAB Function  TreatAsAtomicUnit=on  SystemSampleTime=Ts_MPC
  Memory2 : Memory  InitialCondition=1  InheritSampleTime=on
  Memory3 : Memory  InheritSampleTime=on
  Out1 : Outport
  wires:
  Calibration1/2(i) -> Memory2/1
  Memory2/1 -> Calibration1/2(sample)
  Memory3/1 -> Calibration1/3(data)
  In1/1 -> Calibration1/1(angle)
  Calibration1/1(cal_angle) -> Out1/1
  Calibration1/3(data_out) -> Memory3/1

== system ROPOD_Control_SIM/Subsystem2/Bumper_system/cal4 ==
  In1 : Inport
  Calibration1 : MATLAB Function  TreatAsAtomicUnit=on  SystemSampleTime=Ts_MPC
  Memory2 : Memory  InitialCondition=1  InheritSampleTime=on
  Memory3 : Memory  InheritSampleTime=on
  Out1 : Outport
  wires:
  Calibration1/2(i) -> Memory2/1
  Memory2/1 -> Calibration1/2(sample)
  Memory3/1 -> Calibration1/3(data)
  In1/1 -> Calibration1/1(angle)
  Calibration1/1(cal_angle) -> Out1/1
  Calibration1/3(data_out) -> Memory3/1

== system ROPOD_Control_SIM/Subsystem2/Bumper_system/cal5 ==
  In1 : Inport
  Calibration1 : MATLAB Function  TreatAsAtomicUnit=on  SystemSampleTime=Ts_MPC
  Memory2 : Memory  InitialCondition=1  InheritSampleTime=on
  Memory3 : Memory  InheritSampleTime=on
  Out1 : Outport
  wires:
  Calibration1/3(data_out) -> Memory3/1
  Calibration1/1(cal_angle) -> Out1/1
  In1/1 -> Calibration1/1(angle)
  Memory3/1 -> Calibration1/3(data)
  Memory2/1 -> Calibration1/2(sample)
  Calibration1/2(i) -> Memory2/1

== system ROPOD_Control_SIM/Subsystem2/Bumper_system/cal6 ==
  In1 : Inport
  Calibration1 : MATLAB Function  TreatAsAtomicUnit=on  SystemSampleTime=Ts_MPC
  Memory2 : Memory  InitialCondition=1  InheritSampleTime=on
  Memory3 : Memory  InheritSampleTime=on
  Out1 : Outport
  wires:
  Calibration1/2(i) -> Memory2/1
  Memory2/1 -> Calibration1/2(sample)
  Memory3/1 -> Calibration1/3(data)
  In1/1 -> Calibration1/1(angle)
  Calibration1/1(cal_angle) -> Out1/1
  Calibration1/3(data_out) -> Memory3/1

== system ROPOD_Control_SIM/Subsystem2/Bumper_system/cal7 ==
  In1 : Inport
  Calibration1 : MATLAB Function  TreatAsAtomicUnit=on  SystemSampleTime=Ts_MPC
  Memory2 : Memory  InitialCondition=1  InheritSampleTime=on
  Memory3 : Memory  InheritSampleTime=on
  Out1 : Outport
  wires:
  Calibration1/2(i) -> Memory2/1
  Memory2/1 -> Calibration1/2(sample)
  Memory3/1 -> Calibration1/3(data)
  In1/1 -> Calibration1/1(angle)
  Calibration1/1(cal_angle) -> Out1/1
  Calibration1/3(data_out) -> Memory3/1

== system ROPOD_Control_SIM/Subsystem2/Bumper_system/startup ==
  in : Inport
  Compare To Constant : simulink/Logic and Bit Operations/Compare To Constant  relop=>  const=0.1  OutDataTypeStr=boolean
  Constant : Constant  Value=0
  Digital Clock : DigitalClock  SampleTime=Ts_MPC
  Switch : Switch  Criteria=u2 > Threshold
  out : Outport
  wires:
  Switch/1 -> out/1
  Digital Clock/1 -> Compare To Constant/1
  Compare To Constant/1 -> Switch/2
  in/1 -> Switch/1
  Constant/1 -> Switch/3

== system ROPOD_Control_SIM/Subsystem2/Bumper_system/startup1 ==
  in : Inport
  Compare To Constant : simulink/Logic and Bit Operations/Compare To Constant  relop=>  const=0.1  OutDataTypeStr=boolean
  Constant : Constant  Value=0
  Digital Clock : DigitalClock  SampleTime=Ts_MPC
  Switch : Switch  Criteria=u2 > Threshold
  out : Outport
  wires:
  Switch/1 -> out/1
  Digital Clock/1 -> Compare To Constant/1
  Compare To Constant/1 -> Switch/2
  in/1 -> Switch/1
  Constant/1 -> Switch/3

== system ROPOD_Control_SIM/Subsystem2/Bumper_system/startup2 ==
  in : Inport
  Compare To Constant : simulink/Logic and Bit Operations/Compare To Constant  relop=>  const=0.1  OutDataTypeStr=boolean
  Constant : Constant  Value=0
  Digital Clock : DigitalClock  SampleTime=Ts_MPC
  Switch : Switch  Criteria=u2 > Threshold
  out : Outport
  wires:
  Switch/1 -> out/1
  Digital Clock/1 -> Compare To Constant/1
  Compare To Constant/1 -> Switch/2
  in/1 -> Switch/1
  Constant/1 -> Switch/3

== system ROPOD_Control_SIM/Subsystem2/Bumper_system/startup3 ==
  in : Inport
  Compare To Constant : simulink/Logic and Bit Operations/Compare To Constant  relop=>  const=0.1  OutDataTypeStr=boolean
  Constant : Constant  Value=0
  Digital Clock : DigitalClock  SampleTime=Ts_MPC
  Switch : Switch  Criteria=u2 > Threshold
  out : Outport
  wires:
  Switch/1 -> out/1
  Digital Clock/1 -> Compare To Constant/1
  Compare To Constant/1 -> Switch/2
  in/1 -> Switch/1
  Constant/1 -> Switch/3

== system ROPOD_Control_SIM/FlockController/Flock Velocity controller/G_I_LL_LPF Controller_flock_Theta/Shapeit Integrator (Tustin) ==
  In : Inport
  I_fhz : Inport  Port=2
  reset : Inport  Port=3
  Constant : Constant  Value=0
  Constant4 : Constant
  Constant5 : Constant  Value=0
  Gain2 : Gain  Gain=2*pi
  PID Controller3 : simulink/Continuous/PID Controller  Controller=PID  TimeDomain=Discrete-time  SampleTime=Tsflck  IntegratorMethod=Trapezoidal  FilterMethod=Trapezoidal  Form=Parallel  UseFilter=on  ControllerParametersSource=external  P=0.4  I=0.4*2*pi*3  D=0  N=100  InitialConditionSource=internal  InitialConditionForIntegrator=0  InitialConditionForFilter=0  ExternalReset=level  LimitOutput=on  UpperSaturationLimit=max_ropod_sw_force  LowerSaturationLimit=-max_ropod_sw_force  LinearizeAsGain=on  AntiWindupMode=clamping  Kb=1  TrackingMode=off  Kt=1  PParamMin=[]  PParamMax=[]  IParamMin=[]  IParamMax=[]  DParamMin=[]  DParamMax=[]  NParamMin=[]  NParamMax=[]  KbParamMin=[]  KbParamMax=[]  KtParamMin=[]  KtParamMax=[]  POutMin=[]  POutMax=[]  IOutMin=[]  IOutMax=[]  DOutMin=[]  DOutMax=[]  NOutMin=[]  NOutMax=[]  KbOutMin=[]  KbOutMax=[]  KtOutMin=[]  KtOutMax=[]  IntegratorOutMin=[]  IntegratorOutMax=[]  FilterOutMin=[]  FilterOutMax=[]  SumOutMin=[]  SumOutMax=[]  SumI1OutMin=[]  SumI1OutMax=[]  SumI2OutMin=[]  SumI2OutMax=[]  SumI3OutMin=[]  SumI3OutMax=[]  SumDOutMin=[]  SumDOutMax=[]  SaturationOutMin=[]  SaturationOutMax=[]  IntegratorContinuousStateAttributes=''  IntegratorStateMustResolveToSignalObject=off  IntegratorRTWStateStorageClass=Auto  FilterContinuousStateAttributes=''  FilterStateMustResolveToSignalObject=off  FilterRTWStateStorageClass=Auto  DifferentiatorICPrevScaledInput=0  DifferentiatorOutMin=[]  DifferentiatorOutMax=[]  InitialConditionSetting=State (most efficient)  FilterDiffOutCoefMin=[]  FilterDiffOutCoefMax=[]  SumDenOutMin=[]  SumDenOutMax=[]  SumNumOutMin=[]  SumNumOutMax=[]  ReciprocalOutMin=[]  ReciprocalOutMax=[]  DivideOutMin=[]  DivideOutMax=[]  TunerSelectOption=Transfer Function Based (PID Tuner App)
  Product4 : Product
  Out : Outport
  wires:
  I_fhz/1 -> Product4/2
  Product4/1 -> Gain2/1
  reset/1 -> PID Controller3/6
  Gain2/1 -> PID Controller3/3
  In/1 -> PID Controller3/1
  Constant4/1 -> Product4/1, PID Controller3/2
  Constant5/1 -> PID Controller3/5
  Constant/1 -> PID Controller3/4
  PID Controller3/1 -> Out/1

== system ROPOD_Control_SIM/FlockController/Flock Velocity controller/G_I_LL_LPF Controller_flock_Theta/Shapeit Lead-Lag (Tustin) ==
  In : Inport
  fz : Inport  Port=2
  fp : Inport  Port=3
  Add : Sum  Inputs=+-
  Constant1 : Constant
  Constant2 : Constant  Value=0
  Constant4 : Constant
  Divide : Product  Inputs=*/
  Divide1 : Product  Inputs=/*
  Gain1 : Gain  Gain=2*pi
  Gain2 : Gain  Gain=2*pi
  PID Controller3 : simulink/Continuous/PID Controller  Controller=PID  TimeDomain=Discrete-time  SampleTime=Tsflck  IntegratorMethod=Trapezoidal  FilterMethod=Trapezoidal  Form=Parallel  UseFilter=on  ControllerParametersSource=external  P=0.4  I=0.4*2*pi*3  D=0  N=100  InitialConditionSource=internal  InitialConditionForIntegrator=0  InitialConditionForFilter=0  ExternalReset=none  LimitOutput=off  UpperSaturationLimit=max_hw_tau  LowerSaturationLimit=-max_hw_tau  LinearizeAsGain=on  AntiWindupMode=clamping  Kb=1  TrackingMode=off  Kt=1  PParamMin=[]  PParamMax=[]  IParamMin=[]  IParamMax=[]  DParamMin=[]  DParamMax=[]  NParamMin=[]  NParamMax=[]  KbParamMin=[]  KbParamMax=[]  KtParamMin=[]  KtParamMax=[]  POutMin=[]  POutMax=[]  IOutMin=[]  IOutMax=[]  DOutMin=[]  DOutMax=[]  NOutMin=[]  NOutMax=[]  KbOutMin=[]  KbOutMax=[]  KtOutMin=[]  KtOutMax=[]  IntegratorOutMin=[]  IntegratorOutMax=[]  FilterOutMin=[]  FilterOutMax=[]  SumOutMin=[]  SumOutMax=[]  SumI1OutMin=[]  SumI1OutMax=[]  SumI2OutMin=[]  SumI2OutMax=[]  SumI3OutMin=[]  SumI3OutMax=[]  SumDOutMin=[]  SumDOutMax=[]  SaturationOutMin=[]  SaturationOutMax=[]  IntegratorContinuousStateAttributes=''  IntegratorStateMustResolveToSignalObject=off  IntegratorRTWStateStorageClass=Auto  FilterContinuousStateAttributes=''  FilterStateMustResolveToSignalObject=off  FilterRTWStateStorageClass=Auto  DifferentiatorICPrevScaledInput=0  DifferentiatorOutMin=[]  DifferentiatorOutMax=[]  InitialConditionSetting=State (most efficient)  FilterDiffOutCoefMin=[]  FilterDiffOutCoefMax=[]  SumDenOutMin=[]  SumDenOutMax=[]  SumNumOutMin=[]  SumNumOutMax=[]  ReciprocalOutMin=[]  ReciprocalOutMax=[]  DivideOutMin=[]  DivideOutMax=[]  TunerSelectOption=Transfer Function Based (PID Tuner App)
  Out : Outport
  wires:
  Constant4/1 -> PID Controller3/2
  In/1 -> PID Controller3/1
  PID Controller3/1 -> Out/1
  fz/1 -> Gain2/1
  fp/1 -> Gain1/1
  Gain1/1 -> PID Controller3/5, Divide/2
  Constant2/1 -> PID Controller3/3
  Gain2/1 -> Divide1/1, Divide/1
  Divide/1 -> Add/2
  Constant1/1 -> Add/1
  Add/1 -> Divide1/2
  Divide1/1 -> PID Controller3/4

== system ROPOD_Control_SIM/FlockController/Flock Velocity controller/G_I_LL_LPF Controller_flock_X/Shapeit Integrator (Tustin) ==
  In : Inport
  I_fhz : Inport  Port=2
  reset : Inport  Port=3
  Constant : Constant  Value=0
  Constant4 : Constant
  Constant5 : Constant  Value=0
  Gain2 : Gain  Gain=2*pi
  PID Controller3 : simulink/Continuous/PID Controller  Controller=PID  TimeDomain=Discrete-time  SampleTime=Tsflck  IntegratorMethod=Trapezoidal  FilterMethod=Trapezoidal  Form=Parallel  UseFilter=on  ControllerParametersSource=external  P=0.4  I=0.4*2*pi*3  D=0  N=100  InitialConditionSource=internal  InitialConditionForIntegrator=0  InitialConditionForFilter=0  ExternalReset=level  LimitOutput=on  UpperSaturationLimit=1000  LowerSaturationLimit=-1000  LinearizeAsGain=on  AntiWindupMode=clamping  Kb=1  TrackingMode=off  Kt=1  PParamMin=[]  PParamMax=[]  IParamMin=[]  IParamMax=[]  DParamMin=[]  DParamMax=[]  NParamMin=[]  NParamMax=[]  KbParamMin=[]  KbParamMax=[]  KtParamMin=[]  KtParamMax=[]  POutMin=[]  POutMax=[]  IOutMin=[]  IOutMax=[]  DOutMin=[]  DOutMax=[]  NOutMin=[]  NOutMax=[]  KbOutMin=[]  KbOutMax=[]  KtOutMin=[]  KtOutMax=[]  IntegratorOutMin=[]  IntegratorOutMax=[]  FilterOutMin=[]  FilterOutMax=[]  SumOutMin=[]  SumOutMax=[]  SumI1OutMin=[]  SumI1OutMax=[]  SumI2OutMin=[]  SumI2OutMax=[]  SumI3OutMin=[]  SumI3OutMax=[]  SumDOutMin=[]  SumDOutMax=[]  SaturationOutMin=[]  SaturationOutMax=[]  IntegratorContinuousStateAttributes=''  IntegratorStateMustResolveToSignalObject=off  IntegratorRTWStateStorageClass=Auto  FilterContinuousStateAttributes=''  FilterStateMustResolveToSignalObject=off  FilterRTWStateStorageClass=Auto  DifferentiatorICPrevScaledInput=0  DifferentiatorOutMin=[]  DifferentiatorOutMax=[]  InitialConditionSetting=State (most efficient)  FilterDiffOutCoefMin=[]  FilterDiffOutCoefMax=[]  SumDenOutMin=[]  SumDenOutMax=[]  SumNumOutMin=[]  SumNumOutMax=[]  ReciprocalOutMin=[]  ReciprocalOutMax=[]  DivideOutMin=[]  DivideOutMax=[]  TunerSelectOption=Transfer Function Based (PID Tuner App)
  Product4 : Product
  Out : Outport
  wires:
  I_fhz/1 -> Product4/2
  Product4/1 -> Gain2/1
  reset/1 -> PID Controller3/6
  Gain2/1 -> PID Controller3/3
  In/1 -> PID Controller3/1
  Constant4/1 -> Product4/1, PID Controller3/2
  Constant5/1 -> PID Controller3/5
  Constant/1 -> PID Controller3/4
  PID Controller3/1 -> Out/1

== system ROPOD_Control_SIM/FlockController/Flock Velocity controller/G_I_LL_LPF Controller_flock_X/Shapeit Lead-Lag (Tustin) ==
  In : Inport
  fz : Inport  Port=2
  fp : Inport  Port=3
  Add : Sum  Inputs=+-
  Constant1 : Constant
  Constant2 : Constant  Value=0
  Constant4 : Constant
  Divide : Product  Inputs=*/
  Divide1 : Product  Inputs=/*
  Gain1 : Gain  Gain=2*pi
  Gain2 : Gain  Gain=2*pi
  PID Controller3 : simulink/Continuous/PID Controller  Controller=PID  TimeDomain=Discrete-time  SampleTime=Tsflck  IntegratorMethod=Trapezoidal  FilterMethod=Trapezoidal  Form=Parallel  UseFilter=on  ControllerParametersSource=external  P=0.4  I=0.4*2*pi*3  D=0  N=100  InitialConditionSource=internal  InitialConditionForIntegrator=0  InitialConditionForFilter=0  ExternalReset=none  LimitOutput=off  UpperSaturationLimit=max_hw_tau  LowerSaturationLimit=-max_hw_tau  LinearizeAsGain=on  AntiWindupMode=clamping  Kb=1  TrackingMode=off  Kt=1  PParamMin=[]  PParamMax=[]  IParamMin=[]  IParamMax=[]  DParamMin=[]  DParamMax=[]  NParamMin=[]  NParamMax=[]  KbParamMin=[]  KbParamMax=[]  KtParamMin=[]  KtParamMax=[]  POutMin=[]  POutMax=[]  IOutMin=[]  IOutMax=[]  DOutMin=[]  DOutMax=[]  NOutMin=[]  NOutMax=[]  KbOutMin=[]  KbOutMax=[]  KtOutMin=[]  KtOutMax=[]  IntegratorOutMin=[]  IntegratorOutMax=[]  FilterOutMin=[]  FilterOutMax=[]  SumOutMin=[]  SumOutMax=[]  SumI1OutMin=[]  SumI1OutMax=[]  SumI2OutMin=[]  SumI2OutMax=[]  SumI3OutMin=[]  SumI3OutMax=[]  SumDOutMin=[]  SumDOutMax=[]  SaturationOutMin=[]  SaturationOutMax=[]  IntegratorContinuousStateAttributes=''  IntegratorStateMustResolveToSignalObject=off  IntegratorRTWStateStorageClass=Auto  FilterContinuousStateAttributes=''  FilterStateMustResolveToSignalObject=off  FilterRTWStateStorageClass=Auto  DifferentiatorICPrevScaledInput=0  DifferentiatorOutMin=[]  DifferentiatorOutMax=[]  InitialConditionSetting=State (most efficient)  FilterDiffOutCoefMin=[]  FilterDiffOutCoefMax=[]  SumDenOutMin=[]  SumDenOutMax=[]  SumNumOutMin=[]  SumNumOutMax=[]  ReciprocalOutMin=[]  ReciprocalOutMax=[]  DivideOutMin=[]  DivideOutMax=[]  TunerSelectOption=Transfer Function Based (PID Tuner App)
  Out : Outport
  wires:
  Constant4/1 -> PID Controller3/2
  In/1 -> PID Controller3/1
  PID Controller3/1 -> Out/1
  fz/1 -> Gain2/1
  fp/1 -> Gain1/1
  Gain1/1 -> PID Controller3/5, Divide/2
  Constant2/1 -> PID Controller3/3
  Gain2/1 -> Divide1/1, Divide/1
  Divide/1 -> Add/2
  Constant1/1 -> Add/1
  Add/1 -> Divide1/2
  Divide1/1 -> PID Controller3/4

== system ROPOD_Control_SIM/FlockController/Flock Velocity controller/G_I_LL_LPF Controller_flock_Y/Shapeit Integrator (Tustin) ==
  In : Inport
  I_fhz : Inport  Port=2
  reset : Inport  Port=3
  Constant : Constant  Value=0
  Constant4 : Constant
  Constant5 : Constant  Value=0
  Gain2 : Gain  Gain=2*pi
  PID Controller3 : simulink/Continuous/PID Controller  Controller=PID  TimeDomain=Discrete-time  SampleTime=Tsflck  IntegratorMethod=Trapezoidal  FilterMethod=Trapezoidal  Form=Parallel  UseFilter=on  ControllerParametersSource=external  P=0.4  I=0.4*2*pi*3  D=0  N=100  InitialConditionSource=internal  InitialConditionForIntegrator=0  InitialConditionForFilter=0  ExternalReset=level  LimitOutput=on  UpperSaturationLimit=max_ropod_sw_force  LowerSaturationLimit=-max_ropod_sw_force  LinearizeAsGain=on  AntiWindupMode=clamping  Kb=1  TrackingMode=off  Kt=1  PParamMin=[]  PParamMax=[]  IParamMin=[]  IParamMax=[]  DParamMin=[]  DParamMax=[]  NParamMin=[]  NParamMax=[]  KbParamMin=[]  KbParamMax=[]  KtParamMin=[]  KtParamMax=[]  POutMin=[]  POutMax=[]  IOutMin=[]  IOutMax=[]  DOutMin=[]  DOutMax=[]  NOutMin=[]  NOutMax=[]  KbOutMin=[]  KbOutMax=[]  KtOutMin=[]  KtOutMax=[]  IntegratorOutMin=[]  IntegratorOutMax=[]  FilterOutMin=[]  FilterOutMax=[]  SumOutMin=[]  SumOutMax=[]  SumI1OutMin=[]  SumI1OutMax=[]  SumI2OutMin=[]  SumI2OutMax=[]  SumI3OutMin=[]  SumI3OutMax=[]  SumDOutMin=[]  SumDOutMax=[]  SaturationOutMin=[]  SaturationOutMax=[]  IntegratorContinuousStateAttributes=''  IntegratorStateMustResolveToSignalObject=off  IntegratorRTWStateStorageClass=Auto  FilterContinuousStateAttributes=''  FilterStateMustResolveToSignalObject=off  FilterRTWStateStorageClass=Auto  DifferentiatorICPrevScaledInput=0  DifferentiatorOutMin=[]  DifferentiatorOutMax=[]  InitialConditionSetting=State (most efficient)  FilterDiffOutCoefMin=[]  FilterDiffOutCoefMax=[]  SumDenOutMin=[]  SumDenOutMax=[]  SumNumOutMin=[]  SumNumOutMax=[]  ReciprocalOutMin=[]  ReciprocalOutMax=[]  DivideOutMin=[]  DivideOutMax=[]  TunerSelectOption=Transfer Function Based (PID Tuner App)
  Product4 : Product
  Out : Outport
  wires:
  I_fhz/1 -> Product4/2
  Product4/1 -> Gain2/1
  reset/1 -> PID Controller3/6
  Gain2/1 -> PID Controller3/3
  In/1 -> PID Controller3/1
  Constant4/1 -> Product4/1, PID Controller3/2
  Constant5/1 -> PID Controller3/5
  Constant/1 -> PID Controller3/4
  PID Controller3/1 -> Out/1
